simulink model "RS_DS_CM11_noSimulinkRS"  (R2021b)
settings: Solver=ode1  StartTime=0.0  StopTime=Inf  FixedStep=0.001  RelTol=1e-3  EnableMultiTasking=on
PreLoadFcn:
  | if ~length(which('cmcmd')), cmenv; end
PostLoadFcn:
  | if any(exist('dsrtsu_mdlpostloadfcn', 'file') ~= 0), dsrtsu_mdlpostloadfcn('Execute', bdroot); end
InitFcn:
  | , if any(exist('rtifpga_mdlclblib', 'file') ~= 0), rtifpga_mdlclblib('Init', bdroot); end,
  | , if any(exist('dsmpb_private', 'file') ~= 0), dsmpb_private('dsmpb_mdlclblib', 'Init', bdroot); end,
  | runRS_noSimulinkRS
values from neighbouring files (symbols this model uses):
  RealSimPara = struct    [runRS_SimulinkRS.m]    (also in runRS_noSimulinkRS.m)
libraries: CarMaker4SL x12, simulink x5
(part 2 of 2)

== system RS_DS_CM11_noSimulinkRS/CarMaker/IPG Vehicle/Driver and Drive Cycle/Driver and PI with FF Control ==
  Vehicle_Spd_kph : Inport
  Vehicle_SpdDmd_kph : Inport  Port=2
  Bus Creator : BusCreator  Inputs=6
  Constant : Constant
  Memory1 : Memory
  Memory2 : Memory
  SpdSat : Saturate  UpperLimit=190  LowerLimit=-5
  Vehicle Speed Controller : Subsystem
  km to miles : Gain  Gain=1/1.609344
  DriverBus : Outport
  wires:
  Vehicle Speed Controller/1(AcceleratorPedalPos) -> Bus Creator/2  "AccelPedalCmd"
  Vehicle_SpdDmd_kph/1 -> Memory1/1
  Constant/1 -> Bus Creator/1  "Drive"
  Vehicle Speed Controller/3(BrakeSwitch) -> Bus Creator/4
  SpdSat/1 -> Vehicle Speed Controller/1(RefSpd), km to miles/1, Bus Creator/5  "RefSpd [km/hr]"
  Vehicle Speed Controller/2(BrakePedalPos) -> Bus Creator/3  "BrakePedalCmd"
  Bus Creator/1 -> DriverBus/1  "DriverBus"
  Vehicle_Spd_kph/1 -> Memory2/1
  km to miles/1 -> Bus Creator/6  "RefSpd [mph]"
  Memory1/1 -> SpdSat/1
  Memory2/1 -> Vehicle Speed Controller/2(VehicleSpeed)

== system RS_DS_CM11_noSimulinkRS/CarMaker/IPG Vehicle/CarAndTrailer/CarAndTrailerUpd/CreateBus Brake.IF.In ==
  In : Inport
  BusCreator : BusCreator  Inputs=9
  Demux : Demux  Outputs=9
      settings: DisplayOption=none
  Out : Outport  VectorParamsAs1DForOutWhenUnconnected=off
  wires:
  Demux/9 -> BusCreator/9  "Brake IF Trq_Reg RR"
  Demux/8 -> BusCreator/8  "Brake IF Trq_Reg RL"
  Demux/7 -> BusCreator/7  "Brake IF Trq_Reg FR"
  Demux/6 -> BusCreator/6  "Brake IF Trq_Reg FL"
  Demux/5 -> BusCreator/5  "Brake IF Trq_Reg_max RR"
  Demux/4 -> BusCreator/4  "Brake IF Trq_Reg_max RL"
  Demux/3 -> BusCreator/3  "Brake IF Trq_Reg_max FR"
  Demux/2 -> BusCreator/2  "Brake IF Trq_Reg_max FL"
  Demux/1 -> BusCreator/1  "Brake IF T_env"
  BusCreator/1 -> Out/1
  In/1 -> Demux/1

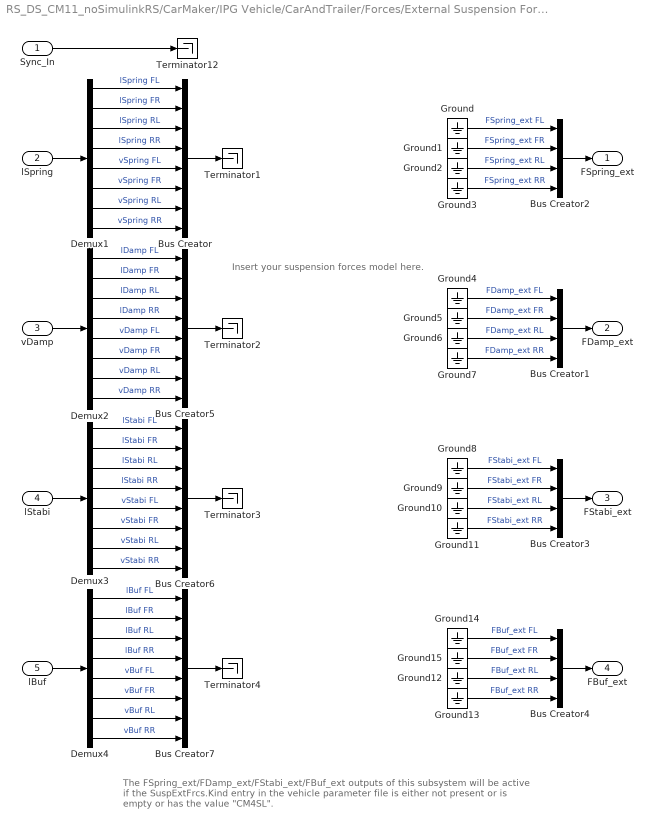
== system RS_DS_CM11_noSimulinkRS/CarMaker/IPG Vehicle/CarAndTrailer/Forces/External Suspension Forces ==
  note: The FSpring_ext/FDamp_ext/FStabi_ext/FBuf_ext outputs of this subsystem will be
      | active if the SuspExtFrcs.Kind entry in the vehicle parameter file
      | is either not present or is empty or has the value "CM4SL".
  note: Insert your suspension forces model here.
  Sync_In : Inport
  lSpring : Inport  Port=2
  vDamp : Inport  Port=3
  lStabi : Inport  Port=4
  lBuf : Inport  Port=5
  Bus Creator{,5..7} (4 alike) : BusCreator  Inputs=8
  Bus Creator{1..4} (4 alike) : BusCreator  Inputs=4
  Demux{1..4} (4 alike) : Demux  Outputs=8
      settings: DisplayOption=none
  Ground{,1..15} (16 alike) : Ground
  Terminator{1..4,12} (5 alike) : Terminator
  FSpring_ext : Outport  VectorParamsAs1DForOutWhenUnconnected=off
  FDamp_ext : Outport  Port=2  VectorParamsAs1DForOutWhenUnconnected=off
  FStabi_ext : Outport  Port=3  VectorParamsAs1DForOutWhenUnconnected=off
  FBuf_ext : Outport  Port=4  VectorParamsAs1DForOutWhenUnconnected=off
  wires:
  Bus Creator7/1 -> Terminator4/1
  Bus Creator6/1 -> Terminator3/1
  Bus Creator5/1 -> Terminator2/1
  Bus Creator/1 -> Terminator1/1
  Demux4/8 -> Bus Creator7/8  "vBuf RR"
  Demux4/7 -> Bus Creator7/7  "vBuf RL"
  Demux4/6 -> Bus Creator7/6  "vBuf FR"
  Demux4/5 -> Bus Creator7/5  "vBuf FL"
  Demux3/8 -> Bus Creator6/8  "vStabi RR"
  Demux3/7 -> Bus Creator6/7  "vStabi RL"
  Demux3/6 -> Bus Creator6/6  "vStabi FR"
  Demux3/5 -> Bus Creator6/5  "vStabi FL"
  Demux2/8 -> Bus Creator5/8  "vDamp RR"
  Demux2/7 -> Bus Creator5/7  "vDamp RL"
  Demux2/6 -> Bus Creator5/6  "vDamp FR"
  Demux2/5 -> Bus Creator5/5  "vDamp FL"
  Demux1/8 -> Bus Creator/8  "vSpring RR"
  Demux1/7 -> Bus Creator/7  "vSpring RL"
  Demux1/6 -> Bus Creator/6  "vSpring FR"
  Demux1/5 -> Bus Creator/5  "vSpring FL"
  Demux2/4 -> Bus Creator5/4  "lDamp RR"
  Demux2/3 -> Bus Creator5/3  "lDamp RL"
  Demux2/2 -> Bus Creator5/2  "lDamp FR"
  Demux2/1 -> Bus Creator5/1  "lDamp FL"
  Demux1/4 -> Bus Creator/4  "lSpring RR"
  Demux1/3 -> Bus Creator/3  "lSpring RL"
  Demux1/2 -> Bus Creator/2  "lSpring FR"
  Demux1/1 -> Bus Creator/1  "lSpring FL"
  Demux3/4 -> Bus Creator6/4  "lStabi RR"
  Demux3/3 -> Bus Creator6/3  "lStabi RL"
  Demux3/2 -> Bus Creator6/2  "lStabi FR"
  Demux3/1 -> Bus Creator6/1  "lStabi FL"
  lStabi/1 -> Demux3/1
  vDamp/1 -> Demux2/1
  lSpring/1 -> Demux1/1
  Demux4/4 -> Bus Creator7/4  "lBuf RR"
  Demux4/3 -> Bus Creator7/3  "lBuf RL"
  Demux4/2 -> Bus Creator7/2  "lBuf FR"
  Demux4/1 -> Bus Creator7/1  "lBuf FL"
  lBuf/1 -> Demux4/1
  Ground14/1 -> Bus Creator4/1  "FBuf_ext FL"
  Ground15/1 -> Bus Creator4/2  "FBuf_ext FR"
  Ground12/1 -> Bus Creator4/3  "FBuf_ext RL"
  Ground13/1 -> Bus Creator4/4  "FBuf_ext RR"
  Bus Creator4/1 -> FBuf_ext/1
  Sync_In/1 -> Terminator12/1
  Bus Creator2/1 -> FSpring_ext/1
  Ground/1 -> Bus Creator2/1  "FSpring_ext FL"
  Ground1/1 -> Bus Creator2/2  "FSpring_ext FR"
  Ground2/1 -> Bus Creator2/3  "FSpring_ext RL"
  Ground3/1 -> Bus Creator2/4  "FSpring_ext RR"
  Ground4/1 -> Bus Creator1/1  "FDamp_ext FL"
  Ground5/1 -> Bus Creator1/2  "FDamp_ext FR"
  Ground6/1 -> Bus Creator1/3  "FDamp_ext RL"
  Ground7/1 -> Bus Creator1/4  "FDamp_ext RR"
  Bus Creator1/1 -> FDamp_ext/1
  Ground8/1 -> Bus Creator3/1  "FStabi_ext FL"
  Ground9/1 -> Bus Creator3/2  "FStabi_ext FR"
  Ground10/1 -> Bus Creator3/3  "FStabi_ext RL"
  Ground11/1 -> Bus Creator3/4  "FStabi_ext RR"
  Bus Creator3/1 -> FStabi_ext/1

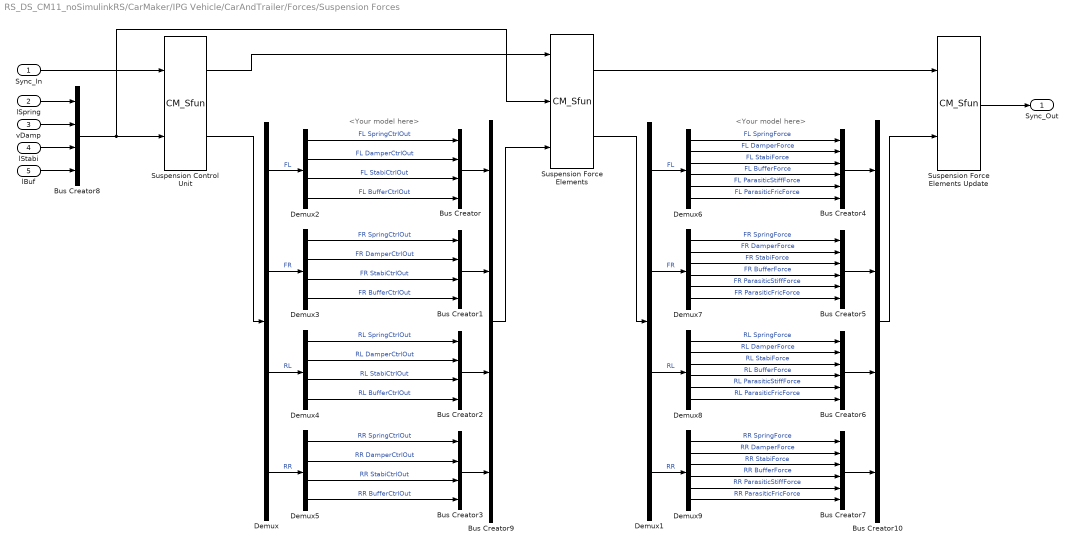
== system RS_DS_CM11_noSimulinkRS/CarMaker/IPG Vehicle/CarAndTrailer/Forces/Suspension Forces ==
  note: <Your model here>
  note: <Your model here>
  Sync_In : Inport
  lSpring : Inport  Port=2
  vDamp : Inport  Port=3
  lStabi : Inport  Port=4
  lBuf : Inport  Port=5
  Bus Creator{,1..3,8..10} (7 alike) : BusCreator  Inputs=4
  Bus Creator{4..7} (4 alike) : BusCreator  Inputs=6
  Demux{,1..5} (6 alike) : Demux
  Demux{6..9} (4 alike) : Demux  Outputs=6
  Suspension Control Unit : S-Function  FunctionName=CM_Sfun  Parameters='ForcesSuspControl'  SFunctionDeploymentMode=off  EnableBusSupport=off
  Suspension Force Elements : S-Function  FunctionName=CM_Sfun  Parameters='ForcesSusp'  SFunctionDeploymentMode=off  EnableBusSupport=off
  Suspension Force Elements Update : S-Function  FunctionName=CM_Sfun  Parameters='ForcesSuspUpd'  SFunctionDeploymentMode=off  EnableBusSupport=off
  Sync_Out : Outport  VectorParamsAs1DForOutWhenUnconnected=off
  wires:
  vDamp/1 -> Bus Creator8/2
  lStabi/1 -> Bus Creator8/3
  lBuf/1 -> Bus Creator8/4
  lSpring/1 -> Bus Creator8/1
  Bus Creator8/1 -> Suspension Control Unit/2, Suspension Force Elements/2
  Sync_In/1 -> Suspension Control Unit/1
  Suspension Control Unit/1 -> Suspension Force Elements/1
  Suspension Force Elements/1 -> Suspension Force Elements Update/1
  Suspension Force Elements Update/1 -> Sync_Out/1
  Bus Creator4/1 -> Bus Creator10/1
  Bus Creator5/1 -> Bus Creator10/2
  Bus Creator6/1 -> Bus Creator10/3
  Bus Creator7/1 -> Bus Creator10/4
  Demux6/1 -> Bus Creator4/1  "FL SpringForce"
  Demux9/1 -> Bus Creator7/1  "RR SpringForce"
  Demux9/2 -> Bus Creator7/2  "RR DamperForce"
  Demux9/3 -> Bus Creator7/3  "RR StabiForce"
  Demux9/4 -> Bus Creator7/4  "RR BufferForce"
  Demux9/5 -> Bus Creator7/5  "RR ParasiticStiffForce"
  Demux9/6 -> Bus Creator7/6  "RR ParasiticFricForce"
  Demux8/1 -> Bus Creator6/1  "RL SpringForce"
  Demux8/2 -> Bus Creator6/2  "RL DamperForce"
  Demux8/4 -> Bus Creator6/4  "RL BufferForce"
  Demux8/5 -> Bus Creator6/5  "RL ParasiticStiffForce"
  Demux8/6 -> Bus Creator6/6  "RL ParasiticFricForce"
  Demux8/3 -> Bus Creator6/3  "RL StabiForce"
  Demux7/1 -> Bus Creator5/1  "FR SpringForce"
  Demux7/2 -> Bus Creator5/2  "FR DamperForce"
  Demux7/3 -> Bus Creator5/3  "FR StabiForce"
  Demux7/4 -> Bus Creator5/4  "FR BufferForce"
  Demux7/5 -> Bus Creator5/5  "FR ParasiticStiffForce"
  Demux7/6 -> Bus Creator5/6  "FR ParasiticFricForce"
  Demux6/2 -> Bus Creator4/2  "FL DamperForce"
  Demux6/3 -> Bus Creator4/3  "FL StabiForce"
  Demux6/4 -> Bus Creator4/4  "FL BufferForce"
  Demux6/5 -> Bus Creator4/5  "FL ParasiticStiffForce"
  Demux6/6 -> Bus Creator4/6  "FL ParasiticFricForce"
  Bus Creator10/1 -> Suspension Force Elements Update/2
  Demux/1 -> Demux2/1  "FL"
  Bus Creator1/1 -> Bus Creator9/2
  Demux/2 -> Demux3/1  "FR"
  Bus Creator2/1 -> Bus Creator9/3
  Demux/3 -> Demux4/1  "RL"
  Bus Creator3/1 -> Bus Creator9/4
  Demux2/1 -> Bus Creator/1  "FL SpringCtrlOut"
  Demux/4 -> Demux5/1  "RR"
  Demux5/1 -> Bus Creator3/1  "RR SpringCtrlOut"
  Demux5/2 -> Bus Creator3/2  "RR DamperCtrlOut"
  Demux5/3 -> Bus Creator3/3  "RR StabiCtrlOut"
  Demux5/4 -> Bus Creator3/4  "RR BufferCtrlOut"
  Demux4/1 -> Bus Creator2/1  "RL SpringCtrlOut"
  Demux4/2 -> Bus Creator2/2  "RL DamperCtrlOut"
  Demux4/4 -> Bus Creator2/4  "RL BufferCtrlOut"
  Demux4/3 -> Bus Creator2/3  "RL StabiCtrlOut"
  Demux3/1 -> Bus Creator1/1  "FR SpringCtrlOut"
  Demux3/2 -> Bus Creator1/2  "FR DamperCtrlOut"
  Demux3/3 -> Bus Creator1/3  "FR StabiCtrlOut"
  Demux3/4 -> Bus Creator1/4  "FR BufferCtrlOut"
  Demux2/2 -> Bus Creator/2  "FL DamperCtrlOut"
  Demux2/3 -> Bus Creator/3  "FL StabiCtrlOut"
  Demux2/4 -> Bus Creator/4  "FL BufferCtrlOut"
  Suspension Control Unit/2 -> Demux/1
  Bus Creator9/1 -> Suspension Force Elements/3
  Bus Creator/1 -> Bus Creator9/1
  Suspension Force Elements/2 -> Demux1/1
  Demux1/1 -> Demux6/1  "FL"
  Demux1/2 -> Demux7/1  "FR"
  Demux1/3 -> Demux8/1  "RL"
  Demux1/4 -> Demux9/1  "RR"

== system RS_DS_CM11_noSimulinkRS/CarMaker/IPG Vehicle/CarAndTrailer/Forces/Tires ==
  note: The TireXX_Out signals will only be used if FileIdent is "CarMaker-Tire-CM4SL" in the tire parameter file!
      | An example parameter file can be found in Data/Tire/DT_CM4SL_UserTire.
  Sync_In : Inport
  TireFL_In : Inport  Port=2
  TireFR_In : Inport  Port=3
  TireRL_In : Inport  Port=4
  TireRR_In : Inport  Port=5
  Bus Creator{1..4} (4 alike) : BusCreator  Inputs=11
  Demux{1..3,8} (4 alike) : Demux  Outputs=7
      settings: DisplayOption=none
  TireFL : Subsystem
  TireFR : Subsystem
  TireRL : Subsystem
  TireRR : Subsystem
  TireFL_Out : Outport  VectorParamsAs1DForOutWhenUnconnected=off
  TireFR_Out : Outport  Port=2  VectorParamsAs1DForOutWhenUnconnected=off
  TireRL_Out : Outport  Port=3  VectorParamsAs1DForOutWhenUnconnected=off
  TireRR_Out : Outport  Port=4  VectorParamsAs1DForOutWhenUnconnected=off
  wires:
  Sync_In/1 -> TireRR/1(Sync_In), TireRL/1(Sync_In), TireFR/1(Sync_In), TireFL/1(Sync_In)
  Bus Creator4/1 -> TireRR_Out/1
  Bus Creator2/1 -> TireRL_Out/1
  Bus Creator1/1 -> TireFR_Out/1
  Demux3/5 -> TireRR/6(Rim_turnv)  "Tire_In Rim_turnv"
  Demux3/4 -> TireRR/5(Rim_rotv)  "Tire_In Rim_rotv"
  Demux3/1 -> TireRR/2(Load)  "Tire_In Load"
  Demux3/7 -> TireRR/8(muRoad)  "Tire_In mu"
  Demux3/6 -> TireRR/7(InclinAngle)  "Tire_In Camber"
  Demux3/2 -> TireRR/3(vxtrans)  "Tire_In vxtrans"
  Demux3/3 -> TireRR/4(vytrans)  "Tire_In vytrans"
  TireRR/11(AlignTrq) -> Bus Creator4/11  "Tire_Out AlignTrq"
  TireRR/10(RollResist) -> Bus Creator4/10  "Tire_Out RollResist"
  TireRR/9(OverturnTrq) -> Bus Creator4/9  "Tire_Out OverturnTrq"
  TireRR/8(LoadFrc) -> Bus Creator4/8  "Tire_Out LoadFrc"
  TireRR/7(SideFrc) -> Bus Creator4/7  "Tire_Out SideFrc"
  TireRR/6(LongFrc) -> Bus Creator4/6  "Tire_Out LongFrc"
  TireRR/5(vBelt) -> Bus Creator4/5  "Tire_Out vBelt"
  TireRR/4(rBelt_eff) -> Bus Creator4/4  "Tire_Out rBelt_eff"
  TireRR/3(TurnSlp) -> Bus Creator4/3  "Tire_Out TurnSlp"
  TireRR/1(Slp) -> Bus Creator4/1  "Tire_Out Slp"
  TireRR/2(Alpha) -> Bus Creator4/2  "Tire_Out Alpha"
  Demux2/5 -> TireRL/6(Rim_turnv)  "Tire_In Rim_turnv"
  Demux2/4 -> TireRL/5(Rim_rotv)  "Tire_In Rim_rotv"
  Demux2/1 -> TireRL/2(Load)  "Tire_In Load"
  Demux2/7 -> TireRL/8(muRoad)  "Tire_In mu"
  Demux2/6 -> TireRL/7(InclinAngle)  "Tire_In Camber"
  Demux2/2 -> TireRL/3(vxtrans)  "Tire_In vxtrans"
  Demux2/3 -> TireRL/4(vytrans)  "Tire_In vytrans"
  TireRL/11(AlignTrq) -> Bus Creator2/11  "Tire_Out AlignTrq"
  TireRL/10(RollResist) -> Bus Creator2/10  "Tire_Out RollResist"
  TireRL/9(OverturnTrq) -> Bus Creator2/9  "Tire_Out OverturnTrq"
  TireRL/8(LoadFrc) -> Bus Creator2/8  "Tire_Out LoadFrc"
  TireRL/7(SideFrc) -> Bus Creator2/7  "Tire_Out SideFrc"
  TireRL/6(LongFrc) -> Bus Creator2/6  "Tire_Out LongFrc"
  TireRL/5(vBelt) -> Bus Creator2/5  "Tire_Out vBelt"
  TireRL/4(rBelt_eff) -> Bus Creator2/4  "Tire_Out rBelt_eff"
  TireRL/3(TurnSlp) -> Bus Creator2/3  "Tire_Out TurnSlp"
  TireRL/1(Slp) -> Bus Creator2/1  "Tire_Out Slp"
  TireRL/2(Alpha) -> Bus Creator2/2  "Tire_Out Alpha"
  Demux1/5 -> TireFR/6(Rim_turnv)  "Tire_In Rim_turnv"
  Demux1/4 -> TireFR/5(Rim_rotv)  "Tire_In Rim_rotv"
  Demux1/1 -> TireFR/2(Load)  "Tire_In Load"
  Demux1/7 -> TireFR/8(muRoad)  "Tire_In mu"
  Demux1/6 -> TireFR/7(InclinAngle)  "Tire_In Camber"
  Demux1/2 -> TireFR/3(vxtrans)  "Tire_In vxtrans"
  Demux1/3 -> TireFR/4(vytrans)  "Tire_In vytrans"
  TireFR/11(AlignTrq) -> Bus Creator1/11  "Tire_Out AlignTrq"
  TireFR/10(RollResist) -> Bus Creator1/10  "Tire_Out RollResist"
  TireFR/9(OverturnTrq) -> Bus Creator1/9  "Tire_Out OverturnTrq"
  TireFR/8(LoadFrc) -> Bus Creator1/8  "Tire_Out LoadFrc"
  TireFR/7(SideFrc) -> Bus Creator1/7  "Tire_Out SideFrc"
  TireFR/6(LongFrc) -> Bus Creator1/6  "Tire_Out LongFrc"
  TireFR/5(vBelt) -> Bus Creator1/5  "Tire_Out vBelt"
  TireFR/4(rBelt_eff) -> Bus Creator1/4  "Tire_Out rBelt_eff"
  TireFR/3(TurnSlp) -> Bus Creator1/3  "Tire_Out TurnSlp"
  TireFR/1(Slp) -> Bus Creator1/1  "Tire_Out Slp"
  TireFR/2(Alpha) -> Bus Creator1/2  "Tire_Out Alpha"
  Demux8/5 -> TireFL/6(Rim_turnv)  "Tire_In Rim_turnv"
  Demux8/4 -> TireFL/5(Rim_rotv)  "Tire_In Rim_rotv"
  TireFL_In/1 -> Demux8/1
  Demux8/1 -> TireFL/2(Load)  "Tire_In Load"
  Demux8/7 -> TireFL/8(muRoad)  "Tire_In mu"
  Demux8/6 -> TireFL/7(InclinAngle)  "Tire_In Camber"
  Demux8/2 -> TireFL/3(vxtrans)  "Tire_In vxtrans"
  Demux8/3 -> TireFL/4(vytrans)  "Tire_In vytrans"
  TireFL/11(AlignTrq) -> Bus Creator3/11  "Tire_Out AlignTrq"
  TireFL/10(RollResist) -> Bus Creator3/10  "Tire_Out RollResist"
  TireFL/9(OverturnTrq) -> Bus Creator3/9  "Tire_Out OverturnTrq"
  TireFL/8(LoadFrc) -> Bus Creator3/8  "Tire_Out LoadFrc"
  TireFL/7(SideFrc) -> Bus Creator3/7  "Tire_Out SideFrc"
  TireFL/6(LongFrc) -> Bus Creator3/6  "Tire_Out LongFrc"
  TireFL/5(vBelt) -> Bus Creator3/5  "Tire_Out vBelt"
  TireFL/4(rBelt_eff) -> Bus Creator3/4  "Tire_Out rBelt_eff"
  TireFL/3(TurnSlp) -> Bus Creator3/3  "Tire_Out TurnSlp"
  TireFL/1(Slp) -> Bus Creator3/1  "Tire_Out Slp"
  TireFL/2(Alpha) -> Bus Creator3/2  "Tire_Out Alpha"
  Bus Creator3/1 -> TireFL_Out/1
  TireFR_In/1 -> Demux1/1
  TireRL_In/1 -> Demux2/1
  TireRR_In/1 -> Demux3/1

== system RS_DS_CM11_noSimulinkRS/CarMaker/IPG Vehicle/CarAndTrailer/Forces/Vehicle Forces ==
  Sync_In : Inport
  Bus Creator1 : BusCreator  Inputs=12
  Bus Creator8 : BusCreator  Inputs=16
  BusCreator1 : BusCreator  Inputs=4
  BusCreator2 : BusCreator  Inputs=9
  Demux : Demux  Outputs=16
      settings: DisplayOption=none
  Demux1 : Demux  Outputs=12
      settings: DisplayOption=none
  Demux2 : Demux  Outputs=13
      settings: DisplayOption=none
  Forces : S-Function  FunctionName=CM_Sfun  Parameters='Forces'  SFunctionDeploymentMode=off  EnableBusSupport=off
  Terminator : Terminator
  Sync_Out : Outport  VectorParamsAs1DForOutWhenUnconnected=off
  Car.Virtual : Outport  Port=2  VectorParamsAs1DForOutWhenUnconnected=off
  Car.Aero : Outport  Port=3  VectorParamsAs1DForOutWhenUnconnected=off
  Car.Load : Outport  Port=4  VectorParamsAs1DForOutWhenUnconnected=off
  wires:
  BusCreator1/1 -> Terminator/1  "Aero IF (in)"
  Demux2/13 -> BusCreator2/9  "car Aero Trq_1 z"
  Demux2/12 -> BusCreator2/8  "car Aero Trq_1 y"
  Demux2/11 -> BusCreator2/7  "car Aero Trq_1 x"
  Demux2/10 -> BusCreator2/6  "car Aero Frc_1 z"
  Demux2/9 -> BusCreator2/5  "car Aero Frc_1 y"
  Demux2/8 -> BusCreator2/4  "car Aero Frc_1 x"
  Demux2/7 -> BusCreator2/3  "car Aero PoA_1 z"
  Demux2/6 -> BusCreator2/2  "car Aero PoA_1 y"
  Demux2/5 -> BusCreator2/1  "car Aero PoA_1 x"
  Demux2/4 -> BusCreator1/4  "car Aero tau_1"
  Demux2/3 -> BusCreator1/3  "car Aero ApproachVel_1 z"
  Demux2/2 -> BusCreator1/2  "car Aero ApproachVel_1 y"
  Demux2/1 -> BusCreator1/1  "car Aero ApproachVel_1 x"
  Demux/16 -> Bus Creator8/16  "Car Load_3 tz"
  Demux/15 -> Bus Creator8/15  "Car Load_3 ty"
  Demux/14 -> Bus Creator8/14  "Car Load_3 tx"
  Demux/13 -> Bus Creator8/13  "Car Load_3 mass"
  Demux1/12 -> Bus Creator1/12  "Car Virtual Trq_0 z"
  Demux1/11 -> Bus Creator1/11  "Car Virtual Trq_0 y"
  Demux1/10 -> Bus Creator1/10  "Car Virtual Trq_0 x"
  Demux1/9 -> Bus Creator1/9  "Car Virtual Trq_1 z"
  Demux1/8 -> Bus Creator1/8  "Car Virtual Trq_1 y"
  Demux1/7 -> Bus Creator1/7  "Car Virtual Trq_1 x"
  Demux1/6 -> Bus Creator1/6  "Car Virtual Frc_0 z"
  Demux1/5 -> Bus Creator1/5  "Car Virtual Frc_0 y"
  Demux1/4 -> Bus Creator1/4  "Car Virtual Frc_0 x"
  Sync_In/1 -> Forces/1
  Forces/1 -> Sync_Out/1
  BusCreator2/1 -> Car.Aero/1
  Demux1/1 -> Bus Creator1/1  "Car Virtual Frc_1 x"
  Demux1/2 -> Bus Creator1/2  "Car Virtual Frc_1 y"
  Demux1/3 -> Bus Creator1/3  "Car Virtual Frc_1 z"
  Forces/3 -> Demux2/1
  Forces/2 -> Demux1/1
  Bus Creator1/1 -> Car.Virtual/1
  Bus Creator8/1 -> Car.Load/1
  Demux/1 -> Bus Creator8/1  "Car Load_0 mass"
  Demux/2 -> Bus Creator8/2  "Car Load_0 tx"
  Demux/3 -> Bus Creator8/3  "Car Load_0 ty"
  Demux/4 -> Bus Creator8/4  "Car Load_0 tz"
  Demux/5 -> Bus Creator8/5  "Car Load_1 mass"
  Demux/6 -> Bus Creator8/6  "Car Load_1 tx"
  Demux/7 -> Bus Creator8/7  "Car Load_1 ty"
  Demux/8 -> Bus Creator8/8  "Car Load_1 tz"
  Demux/9 -> Bus Creator8/9  "Car Load_2 mass"
  Demux/10 -> Bus Creator8/10  "Car Load_2 tx"
  Demux/11 -> Bus Creator8/11  "Car Load_2 ty"
  Demux/12 -> Bus Creator8/12  "Car Load_2 tz"
  Forces/4 -> Demux/1

== system RS_DS_CM11_noSimulinkRS/CarMaker/IPG Vehicle/CarAndTrailer/Trailer/CreateBus Car.Hitch.FrcTrq ==
  In1 : Inport
  Bus Creator7 : BusCreator  Inputs=6
  Demux7 : Demux  Outputs=6
      settings: DisplayOption=none
  Out1 : Outport  VectorParamsAs1DForOutWhenUnconnected=off
  wires:
  In1/1 -> Demux7/1
  Bus Creator7/1 -> Out1/1
  Demux7/6 -> Bus Creator7/6  "Car Hitch Trq2Car z"
  Demux7/5 -> Bus Creator7/5  "Car Hitch Trq2Car y"
  Demux7/4 -> Bus Creator7/4  "Car Hitch Trq2Car x"
  Demux7/3 -> Bus Creator7/3  "Car Hitch Frc2Car z"
  Demux7/2 -> Bus Creator7/2  "Car Hitch Frc2Car y"
  Demux7/1 -> Bus Creator7/1  "Car Hitch Frc2Car x"

== system RS_DS_CM11_noSimulinkRS/CarMaker/IPG Vehicle/CarAndTrailer/Trailer/CreateBus Vhcl.Motion ==
  In1 : Inport
  BusCreator : BusCreator  Inputs=15
  Demux : Demux  Outputs=15
      settings: DisplayOption=none
  Out1 : Outport  VectorParamsAs1DForOutWhenUnconnected=off
  wires:
  Demux/15 -> BusCreator/15  "Vhcl YawAcc"
  Demux/14 -> BusCreator/14  "Vhcl YawVel"
  Demux/13 -> BusCreator/13  "Vhcl Yaw"
  Demux/12 -> BusCreator/12  "Vhcl PitchAcc"
  Demux/11 -> BusCreator/11  "Vhcl PitchVel"
  Demux/10 -> BusCreator/10  "Vhcl Pitch"
  Demux/9 -> BusCreator/9  "Vhcl RollAcc"
  Demux/8 -> BusCreator/8  "Vhcl RollVel"
  Demux/7 -> BusCreator/7  "Vhcl Roll"
  Demux/6 -> BusCreator/6  "Vhcl Hitch_Pos z"
  Demux/5 -> BusCreator/5  "Vhcl Hitch_Pos y"
  Demux/4 -> BusCreator/4  "Vhcl Hitch_Pos x"
  Demux/3 -> BusCreator/3  "Vhcl sRoad"
  Demux/2 -> BusCreator/2  "Vhcl Distance"
  Demux/1 -> BusCreator/1  "Vhcl v"
  In1/1 -> Demux/1
  BusCreator/1 -> Out1/1

== system RS_DS_CM11_noSimulinkRS/CarMaker/IPG Vehicle/CarAndTrailer/Trailer/CreateBus Vhcl.PoI ==
  In1 : Inport
  Bus Creator3 : BusCreator  Inputs=18
  Demux3 : Demux  Outputs=18
      settings: DisplayOption=none
  Out1 : Outport  VectorParamsAs1DForOutWhenUnconnected=off
  wires:
  Demux3/18 -> Bus Creator3/18  "Vhcl PoI_GCS Elev"
  Demux3/17 -> Bus Creator3/17  "Vhcl PoI_GCS Lat"
  Demux3/16 -> Bus Creator3/16  "Vhcl PoI_GCS Long"
  Demux3/15 -> Bus Creator3/15  "Vhcl PoI_Acc_1 z"
  Demux3/14 -> Bus Creator3/14  "Vhcl PoI_Acc_1 y"
  Demux3/13 -> Bus Creator3/13  "Vhcl PoI_Acc_1 x"
  Demux3/12 -> Bus Creator3/12  "Vhcl PoI_Vel_1 z"
  Demux3/11 -> Bus Creator3/11  "Vhcl PoI_Vel_1 y"
  Demux3/10 -> Bus Creator3/10  "Vhcl PoI_Vel_1 x"
  Demux3/9 -> Bus Creator3/9  "Vhcl PoI_Acc z"
  Demux3/8 -> Bus Creator3/8  "Vhcl PoI_Acc y"
  Demux3/7 -> Bus Creator3/7  "Vhcl PoI_Acc x"
  Demux3/6 -> Bus Creator3/6  "Vhcl PoI_Vel z"
  Demux3/5 -> Bus Creator3/5  "Vhcl PoI_Vel y"
  Demux3/4 -> Bus Creator3/4  "Vhcl PoI_Vel x"
  Demux3/3 -> Bus Creator3/3  "Vhcl PoI_Pos z"
  Demux3/2 -> Bus Creator3/2  "Vhcl PoI_Pos y"
  In1/1 -> Demux3/1
  Bus Creator3/1 -> Out1/1
  Demux3/1 -> Bus Creator3/1  "Vhcl PoI_Pos x"

== system RS_DS_CM11_noSimulinkRS/CarMaker/IPG Vehicle/CarAndTrailer/Trailer/CreateBus Vhcl.Steering ==
  In1 : Inport
  Bus Creator3 : BusCreator  Inputs=4
  Demux : Demux
      settings: DisplayOption=none
  Out1 : Outport  VectorParamsAs1DForOutWhenUnconnected=off
  wires:
  Bus Creator3/1 -> Out1/1
  Demux/1 -> Bus Creator3/1  "Vhcl Steering Ang"
  Demux/3 -> Bus Creator3/3  "Vhcl Steering AngAcc"
  Demux/2 -> Bus Creator3/2  "Vhcl Steering AngVel"
  Demux/4 -> Bus Creator3/4  "Vhcl Steering Trq"
  In1/1 -> Demux/1

== system RS_DS_CM11_noSimulinkRS/CarMaker/IPG Vehicle/CarAndTrailer/Trailer/CreateBus Vhcl.Wheel.FL ==
  In1 : Inport
  Bus Creator3 : BusCreator  Inputs=14
  Demux3 : Demux  Outputs=14
      settings: DisplayOption=none
  Out1 : Outport  VectorParamsAs1DForOutWhenUnconnected=off
  wires:
  Demux3/14 -> Bus Creator3/14  "Vhcl Wheel FL Trq_WhlBearing"
  Demux3/13 -> Bus Creator3/13  "Vhcl Wheel FL Trq_T2W"
  Demux3/12 -> Bus Creator3/12  "Vhcl Wheel FL SideSlip"
  Demux3/11 -> Bus Creator3/11  "Vhcl Wheel FL LongSlip"
  Demux3/10 -> Bus Creator3/10  "Vhcl Wheel FL vBelt"
  Demux3/9 -> Bus Creator3/9  "Vhcl Wheel FL Fz"
  Demux3/8 -> Bus Creator3/8  "Vhcl Wheel FL Fy"
  Demux3/7 -> Bus Creator3/7  "Vhcl Wheel FL Fx"
  Demux3/6 -> Bus Creator3/6  "Vhcl Wheel FL r_zxy z"
  Demux3/5 -> Bus Creator3/5  "Vhcl Wheel FL r_zxy y"
  Demux3/4 -> Bus Creator3/4  "Vhcl Wheel FL r_zxy x"
  Demux3/3 -> Bus Creator3/3  "Vhcl Wheel FL t z"
  Demux3/2 -> Bus Creator3/2  "Vhcl Wheel FL t y"
  In1/1 -> Demux3/1
  Bus Creator3/1 -> Out1/1
  Demux3/1 -> Bus Creator3/1  "Vhcl Wheel FL t x"

== system RS_DS_CM11_noSimulinkRS/CarMaker/IPG Vehicle/CarAndTrailer/Trailer/CreateBus Vhcl.Wheel.FR ==
  In1 : Inport
  Bus Creator3 : BusCreator  Inputs=14
  Demux3 : Demux  Outputs=14
      settings: DisplayOption=none
  Out1 : Outport  VectorParamsAs1DForOutWhenUnconnected=off
  wires:
  Demux3/14 -> Bus Creator3/14  "Vhcl Wheel FR Trq_WhlBearing"
  Demux3/13 -> Bus Creator3/13  "Vhcl Wheel FR Trq_T2W"
  Demux3/12 -> Bus Creator3/12  "Vhcl Wheel FR SideSlip"
  Demux3/11 -> Bus Creator3/11  "Vhcl Wheel FR LongSlip"
  Demux3/10 -> Bus Creator3/10  "Vhcl Wheel FR vBelt"
  Demux3/9 -> Bus Creator3/9  "Vhcl Wheel FR Fz"
  Demux3/8 -> Bus Creator3/8  "Vhcl Wheel FR Fy"
  Demux3/7 -> Bus Creator3/7  "Vhcl Wheel FR Fx"
  Demux3/6 -> Bus Creator3/6  "Vhcl Wheel FR r_zxy z"
  Demux3/5 -> Bus Creator3/5  "Vhcl Wheel FR r_zxy y"
  Demux3/4 -> Bus Creator3/4  "Vhcl Wheel FR r_zxy x"
  Demux3/3 -> Bus Creator3/3  "Vhcl Wheel FR t z"
  Demux3/2 -> Bus Creator3/2  "Vhcl Wheel FR t y"
  In1/1 -> Demux3/1
  Bus Creator3/1 -> Out1/1
  Demux3/1 -> Bus Creator3/1  "Vhcl Wheel FR t x"

== system RS_DS_CM11_noSimulinkRS/CarMaker/IPG Vehicle/CarAndTrailer/Trailer/CreateBus Vhcl.Wheel.RL ==
  In1 : Inport
  Bus Creator3 : BusCreator  Inputs=14
  Demux3 : Demux  Outputs=14
      settings: DisplayOption=none
  Out1 : Outport  VectorParamsAs1DForOutWhenUnconnected=off
  wires:
  Demux3/14 -> Bus Creator3/14  "Vhcl Wheel RL Trq_WhlBearing"
  Demux3/13 -> Bus Creator3/13  "Vhcl Wheel RL Trq_T2W"
  Demux3/12 -> Bus Creator3/12  "Vhcl Wheel RL SideSlip"
  Demux3/11 -> Bus Creator3/11  "Vhcl Wheel RL LongSlip"
  Demux3/10 -> Bus Creator3/10  "Vhcl Wheel RL vBelt"
  Demux3/9 -> Bus Creator3/9  "Vhcl Wheel RL Fz"
  Demux3/8 -> Bus Creator3/8  "Vhcl Wheel RL Fy"
  Demux3/7 -> Bus Creator3/7  "Vhcl Wheel RL Fx"
  Demux3/6 -> Bus Creator3/6  "Vhcl Wheel RL r_zxy z"
  Demux3/5 -> Bus Creator3/5  "Vhcl Wheel RL r_zxy y"
  Demux3/4 -> Bus Creator3/4  "Vhcl Wheel RL r_zxy x"
  Demux3/3 -> Bus Creator3/3  "Vhcl Wheel RL t z"
  Demux3/2 -> Bus Creator3/2  "Vhcl Wheel RL t y"
  In1/1 -> Demux3/1
  Bus Creator3/1 -> Out1/1
  Demux3/1 -> Bus Creator3/1  "Vhcl Wheel RL t x"

== system RS_DS_CM11_noSimulinkRS/CarMaker/IPG Vehicle/CarAndTrailer/Trailer/CreateBus Vhcl.Wheel.RR ==
  In1 : Inport
  Bus Creator3 : BusCreator  Inputs=14
  Demux3 : Demux  Outputs=14
      settings: DisplayOption=none
  Out1 : Outport  VectorParamsAs1DForOutWhenUnconnected=off
  wires:
  Demux3/14 -> Bus Creator3/14  "Vhcl Wheel RR Trq_WhlBearing"
  Demux3/13 -> Bus Creator3/13  "Vhcl Wheel RR Trq_T2W"
  Demux3/12 -> Bus Creator3/12  "Vhcl Wheel RR SideSlip"
  Demux3/11 -> Bus Creator3/11  "Vhcl Wheel RR LongSlip"
  Demux3/10 -> Bus Creator3/10  "Vhcl Wheel RR vBelt"
  Demux3/9 -> Bus Creator3/9  "Vhcl Wheel RR Fz"
  Demux3/8 -> Bus Creator3/8  "Vhcl Wheel RR Fy"
  Demux3/7 -> Bus Creator3/7  "Vhcl Wheel RR Fx"
  Demux3/6 -> Bus Creator3/6  "Vhcl Wheel RR r_zxy z"
  Demux3/5 -> Bus Creator3/5  "Vhcl Wheel RR r_zxy y"
  Demux3/4 -> Bus Creator3/4  "Vhcl Wheel RR r_zxy x"
  Demux3/3 -> Bus Creator3/3  "Vhcl Wheel RR t z"
  Demux3/2 -> Bus Creator3/2  "Vhcl Wheel RR t y"
  In1/1 -> Demux3/1
  Bus Creator3/1 -> Out1/1
  Demux3/1 -> Bus Creator3/1  "Vhcl Wheel RR t x"

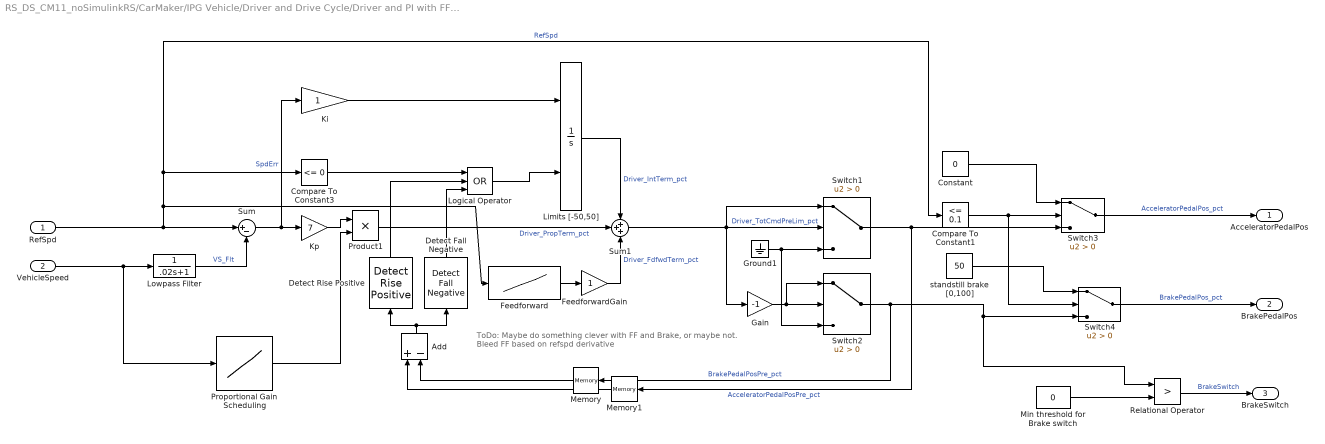
== system RS_DS_CM11_noSimulinkRS/CarMaker/IPG Vehicle/Driver and Drive Cycle/Driver and PI with FF Control/Vehicle Speed Controller ==
  note: ToDo: Maybe do something clever with FF and Brake, or maybe not.
      | Bleed FF based on refspd derivative
  RefSpd : Inport
  VehicleSpeed : Inport  Port=2
  Add : Sum  Inputs=+-
  Compare To Constant1 : simulink/Logic and Bit Operations/Compare To Constant  relop=<=  const=0.1  OutDataTypeStr=boolean  ZeroCross=off
  Compare To Constant3 : simulink/Logic and Bit Operations/Compare To Constant  relop=<=  const=0  OutDataTypeStr=boolean  ZeroCross=off
  Constant : Constant  Value=0
  Detect Fall Negative : simulink/Logic and Bit Operations/Detect Fall Negative  vinit=0  OutDataTypeStr=boolean
      settings: SourceProductBaseCode=SL
  Detect Rise Positive : simulink/Logic and Bit Operations/Detect Rise Positive  vinit=0  OutDataTypeStr=boolean
  Feedforward : Lookup_n-D  NumberOfTableDimensions=1  BreakpointsForDimension1="[0 10    20    30    40    50    60    70    80    90   100   110   120   130   140   150   160]"  Table="[0\t3.5\t12.5\t16\t20\t21\t22\t24.5\t26\t29.5\t32\t33\t34\t36\t37\t38\t39]"  ExtrapMethod=Clip  InternalRulePriority=Speed  RndMeth=Simplest  InputSameDT=on
  FeedforwardGain : Gain
  Gain : Gain  Gain=-1
  Ground1 : Ground
  Ki : Gain
  Kp : Gain  Gain=7
  Limits [-50,50] : Integrator  ExternalReset=either  LimitOutput=on  UpperSaturationLimit=50  LowerSaturationLimit=-50
  Logical Operator : Logic  Operator=OR  Inputs=3  AllPortsSameDT=off  OutDataTypeStr=boolean
  Lowpass Filter : TransferFcn  Denominator=[.02 1]
  Memory : Memory
  Memory1 : Memory
  Min threshold for Brake switch : Constant  Value=0
  Product1 : Product  RndMeth=Zero
  Proportional Gain Scheduling : Lookup_n-D  NumberOfTableDimensions=1  BreakpointsForDimension1=[ 0 30 70]  IndexSearchMethod=Linear search  BeginIndexSearchUsingPreviousIndexResult=on  Table=[1 1 1]  ExtrapMethod=Clip  UseLastTableValue=on  RndMeth=Simplest  InputSameDT=on
  Relational Operator : RelationalOperator  Operator=>  OutDataTypeStr=boolean  RndMeth=Nearest
  Sum : Sum  Inputs=|+-
  Sum1 : Sum  Inputs=+++
  Switch{1..4} (4 alike) : Switch  Criteria=u2 > Threshold
  standstill brake [0,100] : Constant  Value=50
  AcceleratorPedalPos : Outport  VectorParamsAs1DForOutWhenUnconnected=off
  BrakePedalPos : Outport  Port=2  VectorParamsAs1DForOutWhenUnconnected=off
  BrakeSwitch : Outport  Port=3  VectorParamsAs1DForOutWhenUnconnected=off
  wires:
  Kp/1 -> Product1/1
  Min threshold for Brake switch/1 -> Relational Operator/2
  Switch1/1 -> Switch3/3, Memory1/1  "AcceleratorPedalPosPre_pct"
  RefSpd/1 -> Feedforward/1, Compare To Constant1/1, Compare To Constant3/1, Sum/1  "RefSpd"
  Sum/1 -> Kp/1, Ki/1  "SpdErr"
  Limits [-50,50]/1 -> Sum1/1  "Driver_IntTerm_pct"
  VehicleSpeed/1 -> Proportional Gain Scheduling/1, Lowpass Filter/1
  Switch2/1 -> Switch4/3, Relational Operator/1, Memory/1  "BrakePedalPosPre_pct"
  Lowpass Filter/1 -> Sum/2  "VS_Flt"
  Relational Operator/1 -> BrakeSwitch/1  "BrakeSwitch"
  Sum1/1 -> Gain/1, Switch1/1, Switch1/2  "Driver_TotCmdPreLim_pct"
  Ki/1 -> Limits [-50,50]/1
  Ground1/1 -> Switch2/3, Switch1/3
  Gain/1 -> Switch2/1, Switch2/2
  Logical Operator/1 -> Limits [-50,50]/2
  Compare To Constant3/1 -> Logical Operator/1
  Detect Rise Positive/1 -> Logical Operator/2
  Detect Fall Negative/1 -> Logical Operator/3
  Add/1 -> Detect Fall Negative/1, Detect Rise Positive/1
  Memory/1 -> Add/2
  Memory1/1 -> Add/1
  Compare To Constant1/1 -> Switch3/2, Switch4/2
  Switch3/1 -> AcceleratorPedalPos/1  "AcceleratorPedalPos_pct"
  Constant/1 -> Switch3/1
  standstill brake [0,100]/1 -> Switch4/1
  Switch4/1 -> BrakePedalPos/1  "BrakePedalPos_pct"
  Proportional Gain Scheduling/1 -> Product1/2
  Product1/1 -> Sum1/2  "Driver_PropTerm_pct"
  Feedforward/1 -> FeedforwardGain/1
  FeedforwardGain/1 -> Sum1/3  "Driver_FdfwdTerm_pct"

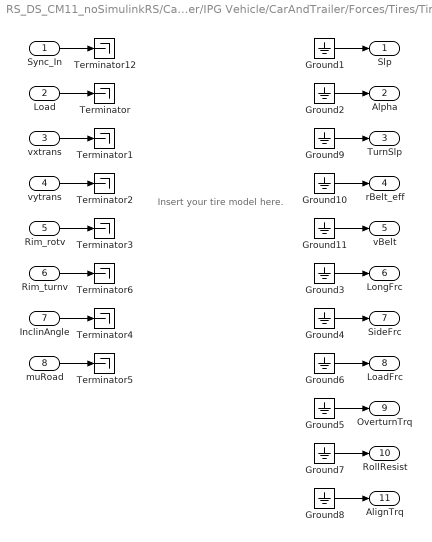
== system RS_DS_CM11_noSimulinkRS/CarMaker/IPG Vehicle/CarAndTrailer/Forces/Tires/TireFL ==
  note: Insert your tire model here.
  Sync_In : Inport
  Load : Inport  Port=2
  vxtrans : Inport  Port=3
  vytrans : Inport  Port=4
  Rim_rotv : Inport  Port=5
  Rim_turnv : Inport  Port=6
  InclinAngle : Inport  Port=7
  muRoad : Inport  Port=8
  Ground{1..11} (11 alike) : Ground
  Terminator{,1..6,12} (8 alike) : Terminator
  Slp : Outport  VectorParamsAs1DForOutWhenUnconnected=off
  Alpha : Outport  Port=2  VectorParamsAs1DForOutWhenUnconnected=off
  TurnSlp : Outport  Port=3  VectorParamsAs1DForOutWhenUnconnected=off
  rBelt_eff : Outport  Port=4  VectorParamsAs1DForOutWhenUnconnected=off
  vBelt : Outport  Port=5  VectorParamsAs1DForOutWhenUnconnected=off
  LongFrc : Outport  Port=6  VectorParamsAs1DForOutWhenUnconnected=off
  SideFrc : Outport  Port=7  VectorParamsAs1DForOutWhenUnconnected=off
  LoadFrc : Outport  Port=8  VectorParamsAs1DForOutWhenUnconnected=off
  OverturnTrq : Outport  Port=9  VectorParamsAs1DForOutWhenUnconnected=off
  RollResist : Outport  Port=10  VectorParamsAs1DForOutWhenUnconnected=off
  AlignTrq : Outport  Port=11  VectorParamsAs1DForOutWhenUnconnected=off
  wires:
  Ground11/1 -> vBelt/1
  Ground10/1 -> rBelt_eff/1
  Ground9/1 -> TurnSlp/1
  Rim_turnv/1 -> Terminator6/1
  Sync_In/1 -> Terminator12/1
  Ground2/1 -> Alpha/1
  Ground3/1 -> LongFrc/1
  Ground4/1 -> SideFrc/1
  Ground5/1 -> OverturnTrq/1
  vxtrans/1 -> Terminator1/1
  vytrans/1 -> Terminator2/1
  Rim_rotv/1 -> Terminator3/1
  InclinAngle/1 -> Terminator4/1
  muRoad/1 -> Terminator5/1
  Load/1 -> Terminator/1
  Ground1/1 -> Slp/1
  Ground6/1 -> LoadFrc/1
  Ground7/1 -> RollResist/1
  Ground8/1 -> AlignTrq/1

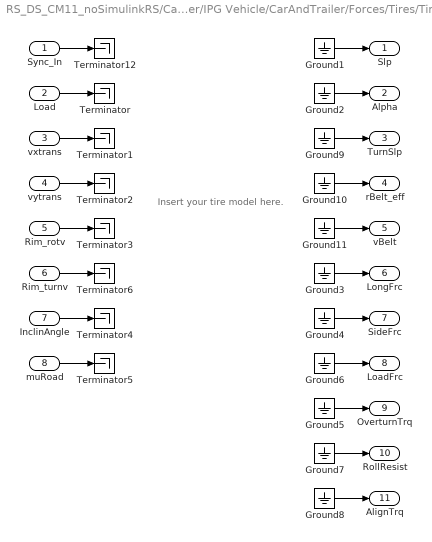
== system RS_DS_CM11_noSimulinkRS/CarMaker/IPG Vehicle/CarAndTrailer/Forces/Tires/TireFR ==
  note: Insert your tire model here.
  Sync_In : Inport
  Load : Inport  Port=2
  vxtrans : Inport  Port=3
  vytrans : Inport  Port=4
  Rim_rotv : Inport  Port=5
  Rim_turnv : Inport  Port=6
  InclinAngle : Inport  Port=7
  muRoad : Inport  Port=8
  Ground{1..11} (11 alike) : Ground
  Terminator{,1..6,12} (8 alike) : Terminator
  Slp : Outport  VectorParamsAs1DForOutWhenUnconnected=off
  Alpha : Outport  Port=2  VectorParamsAs1DForOutWhenUnconnected=off
  TurnSlp : Outport  Port=3  VectorParamsAs1DForOutWhenUnconnected=off
  rBelt_eff : Outport  Port=4  VectorParamsAs1DForOutWhenUnconnected=off
  vBelt : Outport  Port=5  VectorParamsAs1DForOutWhenUnconnected=off
  LongFrc : Outport  Port=6  VectorParamsAs1DForOutWhenUnconnected=off
  SideFrc : Outport  Port=7  VectorParamsAs1DForOutWhenUnconnected=off
  LoadFrc : Outport  Port=8  VectorParamsAs1DForOutWhenUnconnected=off
  OverturnTrq : Outport  Port=9  VectorParamsAs1DForOutWhenUnconnected=off
  RollResist : Outport  Port=10  VectorParamsAs1DForOutWhenUnconnected=off
  AlignTrq : Outport  Port=11  VectorParamsAs1DForOutWhenUnconnected=off
  wires:
  Ground11/1 -> vBelt/1
  Ground10/1 -> rBelt_eff/1
  Ground9/1 -> TurnSlp/1
  Rim_turnv/1 -> Terminator6/1
  Sync_In/1 -> Terminator12/1
  Ground2/1 -> Alpha/1
  Ground3/1 -> LongFrc/1
  Ground4/1 -> SideFrc/1
  Ground5/1 -> OverturnTrq/1
  vxtrans/1 -> Terminator1/1
  vytrans/1 -> Terminator2/1
  Rim_rotv/1 -> Terminator3/1
  InclinAngle/1 -> Terminator4/1
  muRoad/1 -> Terminator5/1
  Load/1 -> Terminator/1
  Ground1/1 -> Slp/1
  Ground6/1 -> LoadFrc/1
  Ground7/1 -> RollResist/1
  Ground8/1 -> AlignTrq/1

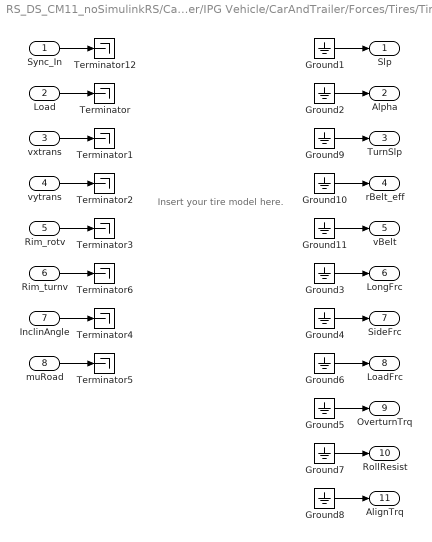
== system RS_DS_CM11_noSimulinkRS/CarMaker/IPG Vehicle/CarAndTrailer/Forces/Tires/TireRL ==
  note: Insert your tire model here.
  Sync_In : Inport
  Load : Inport  Port=2
  vxtrans : Inport  Port=3
  vytrans : Inport  Port=4
  Rim_rotv : Inport  Port=5
  Rim_turnv : Inport  Port=6
  InclinAngle : Inport  Port=7
  muRoad : Inport  Port=8
  Ground{1..11} (11 alike) : Ground
  Terminator{,1..6,12} (8 alike) : Terminator
  Slp : Outport  VectorParamsAs1DForOutWhenUnconnected=off
  Alpha : Outport  Port=2  VectorParamsAs1DForOutWhenUnconnected=off
  TurnSlp : Outport  Port=3  VectorParamsAs1DForOutWhenUnconnected=off
  rBelt_eff : Outport  Port=4  VectorParamsAs1DForOutWhenUnconnected=off
  vBelt : Outport  Port=5  VectorParamsAs1DForOutWhenUnconnected=off
  LongFrc : Outport  Port=6  VectorParamsAs1DForOutWhenUnconnected=off
  SideFrc : Outport  Port=7  VectorParamsAs1DForOutWhenUnconnected=off
  LoadFrc : Outport  Port=8  VectorParamsAs1DForOutWhenUnconnected=off
  OverturnTrq : Outport  Port=9  VectorParamsAs1DForOutWhenUnconnected=off
  RollResist : Outport  Port=10  VectorParamsAs1DForOutWhenUnconnected=off
  AlignTrq : Outport  Port=11  VectorParamsAs1DForOutWhenUnconnected=off
  wires:
  Ground11/1 -> vBelt/1
  Ground10/1 -> rBelt_eff/1
  Ground9/1 -> TurnSlp/1
  Rim_turnv/1 -> Terminator6/1
  Sync_In/1 -> Terminator12/1
  Ground2/1 -> Alpha/1
  Ground3/1 -> LongFrc/1
  Ground4/1 -> SideFrc/1
  Ground5/1 -> OverturnTrq/1
  vxtrans/1 -> Terminator1/1
  vytrans/1 -> Terminator2/1
  Rim_rotv/1 -> Terminator3/1
  InclinAngle/1 -> Terminator4/1
  muRoad/1 -> Terminator5/1
  Load/1 -> Terminator/1
  Ground1/1 -> Slp/1
  Ground6/1 -> LoadFrc/1
  Ground7/1 -> RollResist/1
  Ground8/1 -> AlignTrq/1

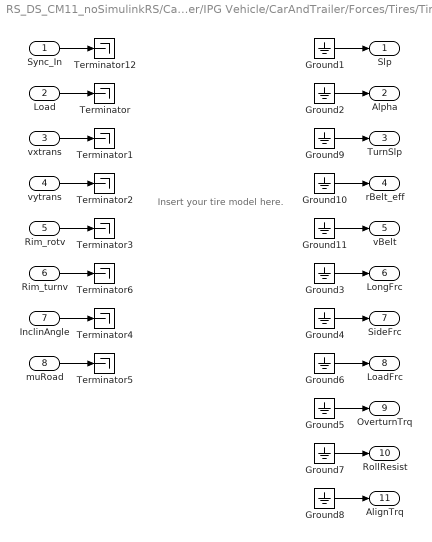
== system RS_DS_CM11_noSimulinkRS/CarMaker/IPG Vehicle/CarAndTrailer/Forces/Tires/TireRR ==
  note: Insert your tire model here.
  Sync_In : Inport
  Load : Inport  Port=2
  vxtrans : Inport  Port=3
  vytrans : Inport  Port=4
  Rim_rotv : Inport  Port=5
  Rim_turnv : Inport  Port=6
  InclinAngle : Inport  Port=7
  muRoad : Inport  Port=8
  Ground{1..11} (11 alike) : Ground
  Terminator{,1..6,12} (8 alike) : Terminator
  Slp : Outport  VectorParamsAs1DForOutWhenUnconnected=off
  Alpha : Outport  Port=2  VectorParamsAs1DForOutWhenUnconnected=off
  TurnSlp : Outport  Port=3  VectorParamsAs1DForOutWhenUnconnected=off
  rBelt_eff : Outport  Port=4  VectorParamsAs1DForOutWhenUnconnected=off
  vBelt : Outport  Port=5  VectorParamsAs1DForOutWhenUnconnected=off
  LongFrc : Outport  Port=6  VectorParamsAs1DForOutWhenUnconnected=off
  SideFrc : Outport  Port=7  VectorParamsAs1DForOutWhenUnconnected=off
  LoadFrc : Outport  Port=8  VectorParamsAs1DForOutWhenUnconnected=off
  OverturnTrq : Outport  Port=9  VectorParamsAs1DForOutWhenUnconnected=off
  RollResist : Outport  Port=10  VectorParamsAs1DForOutWhenUnconnected=off
  AlignTrq : Outport  Port=11  VectorParamsAs1DForOutWhenUnconnected=off
  wires:
  Ground11/1 -> vBelt/1
  Ground10/1 -> rBelt_eff/1
  Ground9/1 -> TurnSlp/1
  Rim_turnv/1 -> Terminator6/1
  Sync_In/1 -> Terminator12/1
  Ground2/1 -> Alpha/1
  Ground3/1 -> LongFrc/1
  Ground4/1 -> SideFrc/1
  Ground5/1 -> OverturnTrq/1
  vxtrans/1 -> Terminator1/1
  vytrans/1 -> Terminator2/1
  Rim_rotv/1 -> Terminator3/1
  InclinAngle/1 -> Terminator4/1
  muRoad/1 -> Terminator5/1
  Load/1 -> Terminator/1
  Ground1/1 -> Slp/1
  Ground6/1 -> LoadFrc/1
  Ground7/1 -> RollResist/1
  Ground8/1 -> AlignTrq/1

== stateflow chart RS_DS_CM11_noSimulinkRS/CarMaker/RealSimHILCycle ==
  state CycleOn
    state InitialWait
      CycleMode=1;
    state RampUp
      CycleMode=2;
      SpeedCmd=SpeedCmd+0.1
    state Driving
      CycleMode=3;
      SpeedCmd=max(SpeedIn, 0)
    state WaitForNextRamp
    InitialWait -> RampUp : after(InitWaitTime,sec)
    (default) -> InitialWait
    RampUp -> Driving [order 1] : [abs(SpeedCmd-SpeedInit)<0.5]
    RampUp -> CycleOn.WaitForNextRamp [order 2] : [abs(SpeedCmd-SpeedInit)>=0.1]
    CycleOn.WaitForNextRamp -> RampUp : after(0.1,sec)
  state Idle
    CycleMode=0;
    SpeedCmd=0;
    CycleTime=0;
  state RampDown
    CycleMode=4;
    SpeedCmd=SpeedCmd-1;
  state WaitForNextRamp
  (default) -> Idle
  Idle -> CycleOn : [SimState>=6 && ...
      | DistanceTravel <= totalDistance && ...
      | SimTime <= totalTime && ...
      | ~RampDownFlag]
  RampDown -> Idle [order 1] : [SpeedCmd<0.5]
  CycleOn -> RampDown : [DistanceTravel > totalDistance || ...
      | SimTime > totalTime || ...
      | RampDownFlag || ...
      | SimState==9]
  WaitForNextRamp -> RampDown : after(0.1,sec)
  RampDown -> WaitForNextRamp [order 2] : [SpeedCmd>=0.5]
  data: SimTime input; SimState input; SpeedIn input; DistanceTravel input; InitWaitTime input; SpeedInit input; totalDistance input; CycleMode output; SpeedCmd output; totalTime input; RampDownFlag input; CycleTime local
